simulink model "modeldefinitiu4t"  (Simulink 7.4)
settings: Solver=ode45  StartTime=t0  StopTime=t1  MaxStep=1e-4
values from neighbouring files (symbols this model uses):
  Ap = 90e3*sqrt(2)/sqrt(3)    [parametres.m]
  E0 = 145e3    (= 145000)    [parametres.m]
  f = 50    [parametres.m]
  ida3 = 0    [parametres.m]
  ida4 = 0    [parametres.m]
  it = [0 0.2 0.200001 0.35 0.3500001 t1]    [parametres.m]
  iv = [0 0 100e6 100e6 0 0]    [parametres.m]
  K3 = 1/20    (= 0.05)    [parametres.m]
  K4 = K3    (= 0.05)    [parametres.m]
  Ki = rl/tau    (= 1140.8)    [parametres.m]
  Kp = Ll/tau    (= 93)    [parametres.m]
  L1 = 0.005    [parametres.m]
  L2 = 0.0025    [parametres.m]
  L3 = 0.004    [parametres.m]
  Lac = 30e-3    (= 0.03)    [parametres.m]
  Ll = Lac    (= 0.03)    [parametres.m]
  Lx = 0.052*0.669    (= 0.034788)    [parametres.m]
  R1 = 0.5    [parametres.m]
  R2 = 0.25    [parametres.m]
  R3 = 0.4    [parametres.m]
  Rac = 3.68/10    (= 0.368)    [parametres.m]
  Rx = 4.8*0.669    (= 3.2112)    [parametres.m]
  sc = 0    [parametres.m]
  T = 1/12e3    (= 8.33333333333e-05)    [parametres.m]
undefined symbols (not defined in the file or in its folder): DiscIntNeverNeededParam
libraries: powerlib x62
(part 1 of 2)
settings Model: Creator=edu  LastModifiedBy=edu

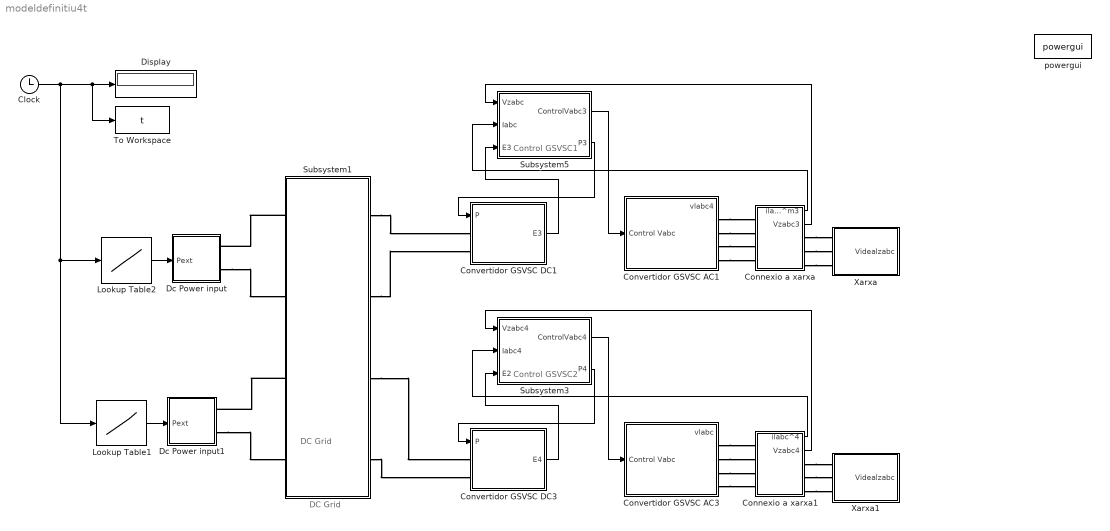
== system modeldefinitiu4t ==
  note: DC Grid
  note: Control GSVSC1
  note: DC Grid
  note: Control GSVSC2
  Clock : Clock
      settings: Decimation=10
  Connexio a xarxa : Subsystem
  Connexio a xarxa1 : Subsystem
  Convertidor GSVSC AC1 : Subsystem
  Convertidor GSVSC AC3 : Subsystem
  Convertidor GSVSC DC1 : Subsystem
  Convertidor GSVSC DC3 : Subsystem
  Dc Power input : Subsystem
  Dc Power input1 : Subsystem
  Display : Display
  Lookup Table1 : Lookup  InputValues=it  Table=iv  OutDataType=fixdt(1, 16)  OutScaling=2^0
  Lookup Table2 : Lookup  InputValues=it  Table=iv  OutDataType=fixdt(1, 16)  OutScaling=2^0
  Subsystem1 : Subsystem
  Subsystem3 : Subsystem
  Subsystem5 : Subsystem
  To Workspace : ToWorkspace  VariableName=t  SampleTime=T  SaveFormat=Array
  Xarxa : Subsystem
  Xarxa1 : Subsystem
  powergui : powerlib/powergui  SystemSampleTime=-1  SimulationMode=Continuous  SampleTime=50e-6  frequency=60  SPID=off  DisableSnubberDevices=off  DisableRonSwitches=off  DisableVfSwitches=off  SwTol=0  Interpol=off  frequencyindice=0  echomessages=off  HookPort=off  DisplayEquations=off  FunctionMessages=off  EnableUseOfTLC=off  x0status=blocks  RestoreLinks=warning  Frange=[0:2:500]  Ylog=off  Xlog=on  ShowGrid=off  save=off  variable=ZData  ZoomFFT=on  StartTime=0.0  cycles=1  DisplayStyle=1  fundamental=60  FreqAxis=off  MaxFrequency=1000  frequencyindicesteady=1  RmsSteady=1  display=off  Ts=0  methode=off
  wires:
  Clock/1 -> Display/1, To Workspace/1, Lookup Table2/1, Lookup Table1/1
  Lookup Table2/1 -> Dc Power input/1(Pext)
  Convertidor GSVSC DC1/1(E3) -> Subsystem5/3(E3)
  Subsystem5/1(ControlVabc3) -> Convertidor GSVSC AC1/1(Control Vabc)
  Connexio a xarxa/1(ilabc^m3) -> Subsystem5/2(Iabc)
  Subsystem5/2(P3) -> Convertidor GSVSC DC1/1(P)
  Connexio a xarxa/2(Vzabc3) -> Subsystem5/1(Vzabc)
  Lookup Table1/1 -> Dc Power input1/1(Pext)
  Convertidor GSVSC DC3/1(E4) -> Subsystem3/3(E2)
  Subsystem3/1(ControlVabc4) -> Convertidor GSVSC AC3/1(Control Vabc)
  Connexio a xarxa1/1(ilabc^4) -> Subsystem3/2(Iabc4)
  Subsystem3/2(P4) -> Convertidor GSVSC DC3/1(P)
  Connexio a xarxa1/2(Vzabc4) -> Subsystem3/1(Vzabc4)
  connections:
  Convertidor GSVSC AC1/RConn2 -- Connexio a xarxa/LConn2
  Connexio a xarxa/RConn1 -- Xarxa/LConn1
  Connexio a xarxa/RConn2 -- Xarxa/LConn2
  Connexio a xarxa/RConn3 -- Xarxa/LConn3
  Subsystem1/LConn1 -- Dc Power input/RConn1
  Dc Power input/RConn2 -- Subsystem1/LConn2
  Subsystem1/RConn2 -- Convertidor GSVSC DC1/LConn2
  Convertidor GSVSC AC1/RConn1 -- Connexio a xarxa/LConn1
  Convertidor GSVSC AC1/RConn3 -- Connexio a xarxa/LConn3
  Convertidor GSVSC AC1/RConn4 -- Connexio a xarxa/LConn4
  Convertidor GSVSC AC3/RConn4 -- Connexio a xarxa1/LConn4
  Convertidor GSVSC AC3/RConn3 -- Connexio a xarxa1/LConn3
  Convertidor GSVSC AC3/RConn1 -- Connexio a xarxa1/LConn1
  Subsystem1/RConn3 -- Convertidor GSVSC DC3/LConn1
  Subsystem1/LConn3 -- Dc Power input1/RConn1
  Connexio a xarxa1/RConn3 -- Xarxa1/LConn3
  Connexio a xarxa1/RConn2 -- Xarxa1/LConn2
  Connexio a xarxa1/RConn1 -- Xarxa1/LConn1
  Convertidor GSVSC AC3/RConn2 -- Connexio a xarxa1/LConn2
  Dc Power input1/RConn2 -- Subsystem1/LConn4
  Subsystem1/RConn4 -- Convertidor GSVSC DC3/LConn2
  Subsystem1/RConn1 -- Convertidor GSVSC DC1/LConn1

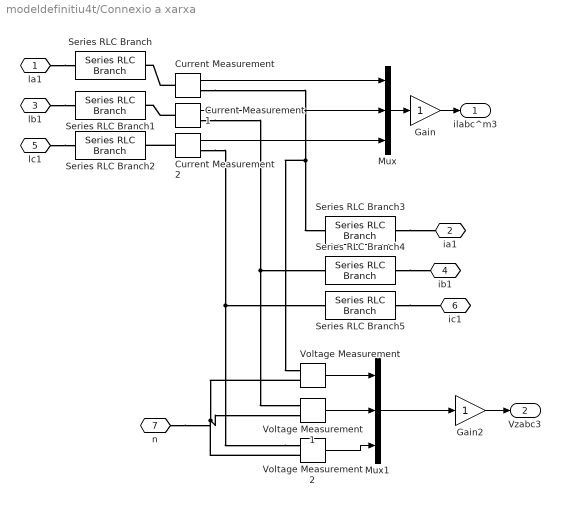
== system modeldefinitiu4t/Connexio a xarxa ==
  Current Measurement : powerlib/Measurements/Current Measurement  DialogController=POWERSYS.PowerSysDialog  SystemSampleTime=-1  PhasorSimulation=off  OutputType=Complex  PSBequivalent=0
  Current Measurement1 : powerlib/Measurements/Current Measurement  DialogController=POWERSYS.PowerSysDialog  SystemSampleTime=-1  PhasorSimulation=off  OutputType=Complex  PSBequivalent=0
  Current Measurement2 : powerlib/Measurements/Current Measurement  DialogController=POWERSYS.PowerSysDialog  SystemSampleTime=-1  PhasorSimulation=off  OutputType=Complex  PSBequivalent=0
  Gain : Gain  ParameterDataType=sfix(16)  ParameterScaling=2^0  OutDataType=sfix(16)  OutScaling=2^0  SampleTime=T
  Gain2 : Gain  ParameterDataType=sfix(16)  ParameterScaling=2^0  OutDataType=sfix(16)  OutScaling=2^0  SampleTime=T
  Mux : Mux  Inputs=3
  Mux1 : Mux  Inputs=3
  Series RLC Branch : powerlib/Elements/Series RLC Branch  DialogController=POWERSYS.PowerSysDialog  PhysicalDomain=powersysdomain  SubClassName=unknown  LeftPortType=p1  RightPortType=p1  LConnTagsString=__new0  RConnTagsString=__new0  BranchType=RL  Resistance=Rac  Inductance=Lac  SetiL0=off  InitialCurrent=0  Capacitance=1e-6  Setx0=off  InitialVoltage=0  Measurements=None
  Series RLC Branch1 : powerlib/Elements/Series RLC Branch  DialogController=POWERSYS.PowerSysDialog  PhysicalDomain=powersysdomain  SubClassName=unknown  LeftPortType=p1  RightPortType=p1  LConnTagsString=__new0  RConnTagsString=__new0  BranchType=RL  Resistance=Rac  Inductance=Lac  SetiL0=off  InitialCurrent=0  Capacitance=1e-6  Setx0=off  InitialVoltage=0  Measurements=None
  Series RLC Branch2 : powerlib/Elements/Series RLC Branch  DialogController=POWERSYS.PowerSysDialog  PhysicalDomain=powersysdomain  SubClassName=unknown  LeftPortType=p1  RightPortType=p1  LConnTagsString=__new0  RConnTagsString=__new0  BranchType=RL  Resistance=Rac  Inductance=Lac  SetiL0=off  InitialCurrent=0  Capacitance=1e-6  Setx0=off  InitialVoltage=0  Measurements=None
  Series RLC Branch3 : powerlib/Elements/Series RLC Branch  DialogController=POWERSYS.PowerSysDialog  PhysicalDomain=powersysdomain  SubClassName=unknown  LeftPortType=p1  RightPortType=p1  LConnTagsString=__new0  RConnTagsString=__new0  BranchType=RL  Resistance=Rx  Inductance=Lx  SetiL0=off  InitialCurrent=0  Capacitance=1e-6  Setx0=off  InitialVoltage=0  Measurements=None
  Series RLC Branch4 : powerlib/Elements/Series RLC Branch  DialogController=POWERSYS.PowerSysDialog  PhysicalDomain=powersysdomain  SubClassName=unknown  LeftPortType=p1  RightPortType=p1  LConnTagsString=__new0  RConnTagsString=__new0  BranchType=RL  Resistance=Rx  Inductance=Lx  SetiL0=off  InitialCurrent=0  Capacitance=1e-6  Setx0=off  InitialVoltage=0  Measurements=None
  Series RLC Branch5 : powerlib/Elements/Series RLC Branch  DialogController=POWERSYS.PowerSysDialog  PhysicalDomain=powersysdomain  SubClassName=unknown  LeftPortType=p1  RightPortType=p1  LConnTagsString=__new0  RConnTagsString=__new0  BranchType=RL  Resistance=Rx  Inductance=Lx  SetiL0=off  InitialCurrent=0  Capacitance=1e-6  Setx0=off  InitialVoltage=0  Measurements=None
  Voltage Measurement : powerlib/Measurements/Voltage Measurement  DialogController=POWERSYS.PowerSysDialog  SystemSampleTime=-1  PhasorSimulation=off  OutputType=Complex  PSBequivalent=0
  Voltage Measurement1 : powerlib/Measurements/Voltage Measurement  DialogController=POWERSYS.PowerSysDialog  SystemSampleTime=-1  PhasorSimulation=off  OutputType=Complex  PSBequivalent=0
  Voltage Measurement2 : powerlib/Measurements/Voltage Measurement  DialogController=POWERSYS.PowerSysDialog  SystemSampleTime=-1  PhasorSimulation=off  OutputType=Complex  PSBequivalent=0
  la1 : PMIOPort  Port=1  Side=Left
  ia1 : PMIOPort  Port=2  Side=Right
  lb1 : PMIOPort  Port=3  Side=Left
  ib1 : PMIOPort  Port=4  Side=Right
  lc1 : PMIOPort  Port=5  Side=Left
  ic1 : PMIOPort  Port=6  Side=Right
  n : PMIOPort  Port=7  Side=Left
  ilabc^m3 : Outport  OutDataType=sfix(16)  OutScaling=2^0
  Vzabc3 : Outport  Port=2
  wires:
  Current Measurement/1 -> Mux/1
  Current Measurement1/1 -> Mux/2
  Current Measurement2/1 -> Mux/3
  Mux/1 -> Gain/1
  Gain/1 -> ilabc^m3/1
  Gain2/1 -> Vzabc3/1
  Voltage Measurement/1 -> Mux1/1
  Voltage Measurement1/1 -> Mux1/2
  Voltage Measurement2/1 -> Mux1/3
  Mux1/1 -> Gain2/1
  connections:
  la1/RConn1 -- Series RLC Branch/LConn1
  Current Measurement/LConn1 -- Series RLC Branch/RConn1
  lb1/RConn1 -- Series RLC Branch1/LConn1
  Current Measurement1/LConn1 -- Series RLC Branch1/RConn1
  lc1/RConn1 -- Series RLC Branch2/LConn1
  Current Measurement2/LConn1 -- Series RLC Branch2/RConn1
  Voltage Measurement2/LConn1 -- Current Measurement2/RConn1 -- Series RLC Branch5/LConn1
  Current Measurement1/RConn1 -- Series RLC Branch4/LConn1 -- Voltage Measurement1/LConn1
  Current Measurement/RConn1 -- Series RLC Branch3/LConn1 -- Voltage Measurement/LConn1
  Series RLC Branch3/RConn1 -- ia1/RConn1
  Series RLC Branch4/RConn1 -- ib1/RConn1
  Series RLC Branch5/RConn1 -- ic1/RConn1
  Voltage Measurement2/LConn2 -- Voltage Measurement/LConn2 -- Voltage Measurement1/LConn2 -- n/RConn1

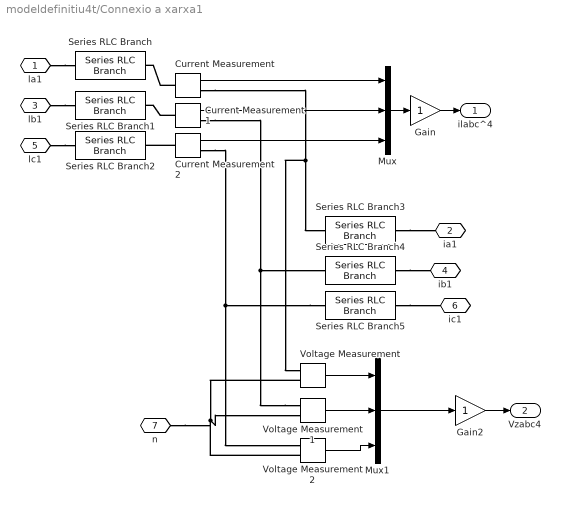
== system modeldefinitiu4t/Connexio a xarxa1 ==
  Current Measurement : powerlib/Measurements/Current Measurement  DialogController=POWERSYS.PowerSysDialog  SystemSampleTime=-1  PhasorSimulation=off  OutputType=Complex  PSBequivalent=0
  Current Measurement1 : powerlib/Measurements/Current Measurement  DialogController=POWERSYS.PowerSysDialog  SystemSampleTime=-1  PhasorSimulation=off  OutputType=Complex  PSBequivalent=0
  Current Measurement2 : powerlib/Measurements/Current Measurement  DialogController=POWERSYS.PowerSysDialog  SystemSampleTime=-1  PhasorSimulation=off  OutputType=Complex  PSBequivalent=0
  Gain : Gain  ParameterDataType=sfix(16)  ParameterScaling=2^0  OutDataType=sfix(16)  OutScaling=2^0  SampleTime=T
  Gain2 : Gain  ParameterDataType=sfix(16)  ParameterScaling=2^0  OutDataType=sfix(16)  OutScaling=2^0  SampleTime=T
  Mux : Mux  Inputs=3
  Mux1 : Mux  Inputs=3
  Series RLC Branch : powerlib/Elements/Series RLC Branch  DialogController=POWERSYS.PowerSysDialog  PhysicalDomain=powersysdomain  SubClassName=unknown  LeftPortType=p1  RightPortType=p1  LConnTagsString=__new0  RConnTagsString=__new0  BranchType=RL  Resistance=Rac  Inductance=Lac  SetiL0=off  InitialCurrent=0  Capacitance=1e-6  Setx0=off  InitialVoltage=0  Measurements=None
  Series RLC Branch1 : powerlib/Elements/Series RLC Branch  DialogController=POWERSYS.PowerSysDialog  PhysicalDomain=powersysdomain  SubClassName=unknown  LeftPortType=p1  RightPortType=p1  LConnTagsString=__new0  RConnTagsString=__new0  BranchType=RL  Resistance=Rac  Inductance=Lac  SetiL0=off  InitialCurrent=0  Capacitance=1e-6  Setx0=off  InitialVoltage=0  Measurements=None
  Series RLC Branch2 : powerlib/Elements/Series RLC Branch  DialogController=POWERSYS.PowerSysDialog  PhysicalDomain=powersysdomain  SubClassName=unknown  LeftPortType=p1  RightPortType=p1  LConnTagsString=__new0  RConnTagsString=__new0  BranchType=RL  Resistance=Rac  Inductance=Lac  SetiL0=off  InitialCurrent=0  Capacitance=1e-6  Setx0=off  InitialVoltage=0  Measurements=None
  Series RLC Branch3 : powerlib/Elements/Series RLC Branch  DialogController=POWERSYS.PowerSysDialog  PhysicalDomain=powersysdomain  SubClassName=unknown  LeftPortType=p1  RightPortType=p1  LConnTagsString=__new0  RConnTagsString=__new0  BranchType=RL  Resistance=Rx  Inductance=Lx  SetiL0=off  InitialCurrent=0  Capacitance=1e-6  Setx0=off  InitialVoltage=0  Measurements=None
  Series RLC Branch4 : powerlib/Elements/Series RLC Branch  DialogController=POWERSYS.PowerSysDialog  PhysicalDomain=powersysdomain  SubClassName=unknown  LeftPortType=p1  RightPortType=p1  LConnTagsString=__new0  RConnTagsString=__new0  BranchType=RL  Resistance=Rx  Inductance=Lx  SetiL0=off  InitialCurrent=0  Capacitance=1e-6  Setx0=off  InitialVoltage=0  Measurements=None
  Series RLC Branch5 : powerlib/Elements/Series RLC Branch  DialogController=POWERSYS.PowerSysDialog  PhysicalDomain=powersysdomain  SubClassName=unknown  LeftPortType=p1  RightPortType=p1  LConnTagsString=__new0  RConnTagsString=__new0  BranchType=RL  Resistance=Rx  Inductance=Lx  SetiL0=off  InitialCurrent=0  Capacitance=1e-6  Setx0=off  InitialVoltage=0  Measurements=None
  Voltage Measurement : powerlib/Measurements/Voltage Measurement  DialogController=POWERSYS.PowerSysDialog  SystemSampleTime=-1  PhasorSimulation=off  OutputType=Complex  PSBequivalent=0
  Voltage Measurement1 : powerlib/Measurements/Voltage Measurement  DialogController=POWERSYS.PowerSysDialog  SystemSampleTime=-1  PhasorSimulation=off  OutputType=Complex  PSBequivalent=0
  Voltage Measurement2 : powerlib/Measurements/Voltage Measurement  DialogController=POWERSYS.PowerSysDialog  SystemSampleTime=-1  PhasorSimulation=off  OutputType=Complex  PSBequivalent=0
  la1 : PMIOPort  Port=1  Side=Left
  ia1 : PMIOPort  Port=2  Side=Right
  lb1 : PMIOPort  Port=3  Side=Left
  ib1 : PMIOPort  Port=4  Side=Right
  lc1 : PMIOPort  Port=5  Side=Left
  ic1 : PMIOPort  Port=6  Side=Right
  n : PMIOPort  Port=7  Side=Left
  ilabc^4 : Outport  OutDataType=sfix(16)  OutScaling=2^0
  Vzabc4 : Outport  Port=2
  wires:
  Mux1/1 -> Gain2/1
  Voltage Measurement2/1 -> Mux1/3
  Voltage Measurement1/1 -> Mux1/2
  Voltage Measurement/1 -> Mux1/1
  Gain2/1 -> Vzabc4/1
  Gain/1 -> ilabc^4/1
  Mux/1 -> Gain/1
  Current Measurement2/1 -> Mux/3
  Current Measurement1/1 -> Mux/2
  Current Measurement/1 -> Mux/1
  connections:
  n/RConn1 -- Voltage Measurement1/LConn2 -- Voltage Measurement/LConn2 -- Voltage Measurement2/LConn2
  Series RLC Branch5/RConn1 -- ic1/RConn1
  Series RLC Branch4/RConn1 -- ib1/RConn1
  Series RLC Branch3/RConn1 -- ia1/RConn1
  Voltage Measurement/LConn1 -- Series RLC Branch3/LConn1 -- Current Measurement/RConn1
  Voltage Measurement1/LConn1 -- Series RLC Branch4/LConn1 -- Current Measurement1/RConn1
  Series RLC Branch5/LConn1 -- Current Measurement2/RConn1 -- Voltage Measurement2/LConn1
  Current Measurement2/LConn1 -- Series RLC Branch2/RConn1
  lc1/RConn1 -- Series RLC Branch2/LConn1
  Current Measurement1/LConn1 -- Series RLC Branch1/RConn1
  lb1/RConn1 -- Series RLC Branch1/LConn1
  Current Measurement/LConn1 -- Series RLC Branch/RConn1
  la1/RConn1 -- Series RLC Branch/LConn1

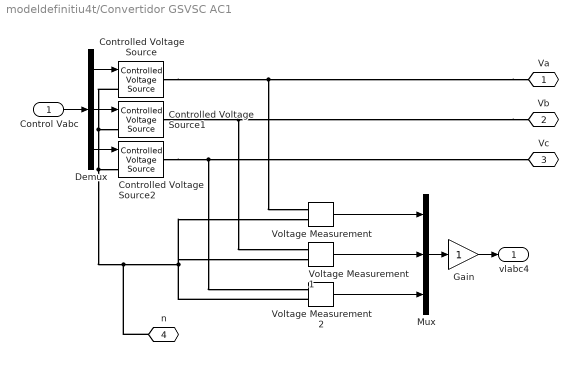
== system modeldefinitiu4t/Convertidor GSVSC AC1 ==
  Control Vabc : Inport
  Controlled Voltage Source : powerlib/Electrical Sources/Controlled Voltage Source  DialogController=POWERSYS.PowerSysDialog  SystemSampleTime=-1  Initialize=on  Source_Type=AC  Amplitude=0  Phase=0  Frequency=0  Measurements=None
  Controlled Voltage Source1 : powerlib/Electrical Sources/Controlled Voltage Source  DialogController=POWERSYS.PowerSysDialog  SystemSampleTime=-1  Initialize=on  Source_Type=AC  Amplitude=0  Phase=0  Frequency=0  Measurements=None
  Controlled Voltage Source2 : powerlib/Electrical Sources/Controlled Voltage Source  DialogController=POWERSYS.PowerSysDialog  SystemSampleTime=-1  Initialize=on  Source_Type=AC  Amplitude=0  Phase=0  Frequency=0  Measurements=None
  Demux : Demux  Outputs=3
  Gain : Gain  ParameterDataType=sfix(16)  ParameterScaling=2^0  OutDataType=sfix(16)  OutScaling=2^0  SampleTime=T
  Mux : Mux  Inputs=3
  Voltage Measurement : powerlib/Measurements/Voltage Measurement  DialogController=POWERSYS.PowerSysDialog  SystemSampleTime=-1  PhasorSimulation=off  OutputType=Complex  PSBequivalent=0
  Voltage Measurement1 : powerlib/Measurements/Voltage Measurement  DialogController=POWERSYS.PowerSysDialog  SystemSampleTime=-1  PhasorSimulation=off  OutputType=Complex  PSBequivalent=0
  Voltage Measurement2 : powerlib/Measurements/Voltage Measurement  DialogController=POWERSYS.PowerSysDialog  SystemSampleTime=-1  PhasorSimulation=off  OutputType=Complex  PSBequivalent=0
  Va : PMIOPort  Port=1  Side=Right
  Vb : PMIOPort  Port=2  Side=Right
  Vc : PMIOPort  Port=3  Side=Right
  n : PMIOPort  Port=4  Side=Right
  vlabc4 : Outport
  wires:
  Demux/3 -> Controlled Voltage Source2/1
  Demux/2 -> Controlled Voltage Source1/1
  Demux/1 -> Controlled Voltage Source/1
  Voltage Measurement/1 -> Mux/1
  Voltage Measurement1/1 -> Mux/2
  Voltage Measurement2/1 -> Mux/3
  Mux/1 -> Gain/1
  Gain/1 -> vlabc4/1
  Control Vabc/1 -> Demux/1
  connections:
  Va/RConn1 -- Controlled Voltage Source/RConn1 -- Voltage Measurement/LConn1
  Vb/RConn1 -- Controlled Voltage Source1/RConn1 -- Voltage Measurement1/LConn1
  Controlled Voltage Source2/RConn1 -- Vc/RConn1 -- Voltage Measurement2/LConn1
  Controlled Voltage Source/LConn1 -- Controlled Voltage Source1/LConn1 -- Controlled Voltage Source2/LConn1 -- Voltage Measurement2/LConn2 -- Voltage Measurement/LConn2 -- Voltage Measurement1/LConn2 -- n/RConn1

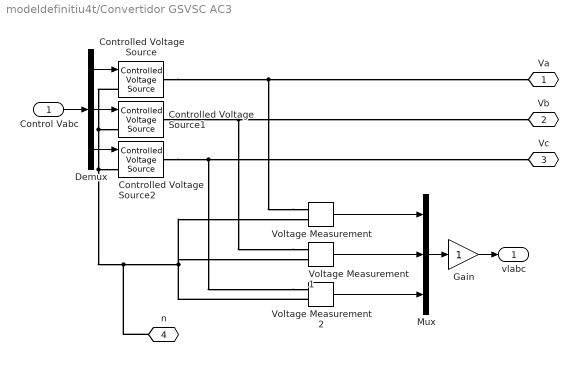
== system modeldefinitiu4t/Convertidor GSVSC AC3 ==
  Control Vabc : Inport
  Controlled Voltage Source : powerlib/Electrical Sources/Controlled Voltage Source  DialogController=POWERSYS.PowerSysDialog  SystemSampleTime=-1  Initialize=on  Source_Type=AC  Amplitude=0  Phase=0  Frequency=0  Measurements=None
  Controlled Voltage Source1 : powerlib/Electrical Sources/Controlled Voltage Source  DialogController=POWERSYS.PowerSysDialog  SystemSampleTime=-1  Initialize=on  Source_Type=AC  Amplitude=0  Phase=0  Frequency=0  Measurements=None
  Controlled Voltage Source2 : powerlib/Electrical Sources/Controlled Voltage Source  DialogController=POWERSYS.PowerSysDialog  SystemSampleTime=-1  Initialize=on  Source_Type=AC  Amplitude=0  Phase=0  Frequency=0  Measurements=None
  Demux : Demux  Outputs=3
  Gain : Gain  ParameterDataType=sfix(16)  ParameterScaling=2^0  OutDataType=sfix(16)  OutScaling=2^0  SampleTime=T
  Mux : Mux  Inputs=3
  Voltage Measurement : powerlib/Measurements/Voltage Measurement  DialogController=POWERSYS.PowerSysDialog  SystemSampleTime=-1  PhasorSimulation=off  OutputType=Complex  PSBequivalent=0
  Voltage Measurement1 : powerlib/Measurements/Voltage Measurement  DialogController=POWERSYS.PowerSysDialog  SystemSampleTime=-1  PhasorSimulation=off  OutputType=Complex  PSBequivalent=0
  Voltage Measurement2 : powerlib/Measurements/Voltage Measurement  DialogController=POWERSYS.PowerSysDialog  SystemSampleTime=-1  PhasorSimulation=off  OutputType=Complex  PSBequivalent=0
  Va : PMIOPort  Port=1  Side=Right
  Vb : PMIOPort  Port=2  Side=Right
  Vc : PMIOPort  Port=3  Side=Right
  n : PMIOPort  Port=4  Side=Right
  vlabc : Outport
  wires:
  Control Vabc/1 -> Demux/1
  Gain/1 -> vlabc/1
  Mux/1 -> Gain/1
  Voltage Measurement2/1 -> Mux/3
  Voltage Measurement1/1 -> Mux/2
  Voltage Measurement/1 -> Mux/1
  Demux/1 -> Controlled Voltage Source/1
  Demux/2 -> Controlled Voltage Source1/1
  Demux/3 -> Controlled Voltage Source2/1
  connections:
  n/RConn1 -- Voltage Measurement1/LConn2 -- Voltage Measurement/LConn2 -- Voltage Measurement2/LConn2 -- Controlled Voltage Source2/LConn1 -- Controlled Voltage Source1/LConn1 -- Controlled Voltage Source/LConn1
  Voltage Measurement2/LConn1 -- Vc/RConn1 -- Controlled Voltage Source2/RConn1
  Voltage Measurement1/LConn1 -- Controlled Voltage Source1/RConn1 -- Vb/RConn1
  Voltage Measurement/LConn1 -- Controlled Voltage Source/RConn1 -- Va/RConn1

== system modeldefinitiu4t/Convertidor GSVSC DC1 ==
  P : Inport
  Controlled Current Source1 : powerlib/Electrical Sources/Controlled Current Source  DialogController=POWERSYS.PowerSysDialog  SystemSampleTime=-1  Initialize=on  Source_Type=DC  Amplitude=10  Phase=0  Frequency=0  Measurements=None
  Current Measurement1 : powerlib/Measurements/Current Measurement  DialogController=POWERSYS.PowerSysDialog  SystemSampleTime=-1  PhasorSimulation=off  OutputType=Complex  PSBequivalent=0
  Divide : Product  Inputs=/*  OutDataType=fixdt(1, 16)  OutScaling=2^-10
  Gain1 : Gain  ParameterDataType=sfix(16)  ParameterScaling=2^0  OutDataType=sfix(16)  OutScaling=2^0  SampleTime=T
  Gain2 : Gain  ParameterDataType=sfix(16)  ParameterScaling=2^0  OutDataType=sfix(16)  OutScaling=2^0  SampleTime=T
  Scope : Scope
      settings: YMin=-100  YMax=700
  To Workspace1 : ToWorkspace  VariableName=i3  SampleTime=-1  SaveFormat=Array
  To Workspace2 : ToWorkspace  VariableName=E3  SampleTime=-1  SaveFormat=Array
  Voltage Measurement : powerlib/Measurements/Voltage Measurement  DialogController=POWERSYS.PowerSysDialog  SystemSampleTime=-1  PhasorSimulation=off  OutputType=Complex  PSBequivalent=0
  Idc+ : PMIOPort  Port=1  Side=Left
  idc- : PMIOPort  Port=2  Side=Left
  E3 : Outport
  wires:
  Voltage Measurement/1 -> E3/1, Divide/1, Gain1/1
  Divide/1 -> Controlled Current Source1/1
  Current Measurement1/1 -> Gain2/1
  P/1 -> Divide/2
  Gain1/1 -> To Workspace2/1
  Gain2/1 -> To Workspace1/1, Scope/1
  connections:
  Idc+/RConn1 -- Controlled Current Source1/LConn1 -- Voltage Measurement/LConn1
  Current Measurement1/LConn1 -- Controlled Current Source1/RConn1
  Current Measurement1/RConn1 -- idc-/RConn1 -- Voltage Measurement/LConn2

== system modeldefinitiu4t/Convertidor GSVSC DC3 ==
  P : Inport
  Controlled Current Source1 : powerlib/Electrical Sources/Controlled Current Source  DialogController=POWERSYS.PowerSysDialog  SystemSampleTime=-1  Initialize=on  Source_Type=DC  Amplitude=10  Phase=0  Frequency=0  Measurements=None
  Current Measurement1 : powerlib/Measurements/Current Measurement  DialogController=POWERSYS.PowerSysDialog  SystemSampleTime=-1  PhasorSimulation=off  OutputType=Complex  PSBequivalent=0
  Divide : Product  Inputs=/*  OutDataType=fixdt(1, 16)  OutScaling=2^-10
  Gain1 : Gain  ParameterDataType=sfix(16)  ParameterScaling=2^0  OutDataType=sfix(16)  OutScaling=2^0  SampleTime=T
  Gain2 : Gain  ParameterDataType=sfix(16)  ParameterScaling=2^0  OutDataType=sfix(16)  OutScaling=2^0  SampleTime=T
  Scope : Scope
      settings: YMin=-100  YMax=700
  To Workspace1 : ToWorkspace  VariableName=i4  SampleTime=-1  SaveFormat=Array
  To Workspace2 : ToWorkspace  VariableName=E4  SampleTime=-1  SaveFormat=Array
  Voltage Measurement : powerlib/Measurements/Voltage Measurement  DialogController=POWERSYS.PowerSysDialog  SystemSampleTime=-1  PhasorSimulation=off  OutputType=Complex  PSBequivalent=0
  Idc+ : PMIOPort  Port=1  Side=Left
  idc- : PMIOPort  Port=2  Side=Left
  E4 : Outport
  wires:
  Gain2/1 -> Scope/1, To Workspace1/1
  Gain1/1 -> To Workspace2/1
  P/1 -> Divide/2
  Current Measurement1/1 -> Gain2/1
  Divide/1 -> Controlled Current Source1/1
  Voltage Measurement/1 -> Gain1/1, Divide/1, E4/1
  connections:
  Voltage Measurement/LConn2 -- idc-/RConn1 -- Current Measurement1/RConn1
  Current Measurement1/LConn1 -- Controlled Current Source1/RConn1
  Voltage Measurement/LConn1 -- Controlled Current Source1/LConn1 -- Idc+/RConn1

== system modeldefinitiu4t/Dc Power input ==
  Pext : Inport
  Controlled Current Source2 : powerlib/Electrical Sources/Controlled Current Source  DialogController=POWERSYS.PowerSysDialog  SystemSampleTime=-1  Initialize=on  Source_Type=DC  Amplitude=10  Phase=0  Frequency=0  Measurements=None
  Current Measurement1 : powerlib/Measurements/Current Measurement  DialogController=POWERSYS.PowerSysDialog  SystemSampleTime=-1  PhasorSimulation=off  OutputType=Complex  PSBequivalent=0
  Divide1 : Product  Inputs=*/  OutDataType=fixdt(1, 16)  OutScaling=2^-10
  Gain1 : Gain  ParameterDataType=sfix(16)  ParameterScaling=2^0  OutDataType=sfix(16)  OutScaling=2^0  SampleTime=T
  Gain2 : Gain  ParameterDataType=sfix(16)  ParameterScaling=2^0  OutDataType=sfix(16)  OutScaling=2^0  SampleTime=T
  Gain3 : Gain  ParameterDataType=sfix(16)  ParameterScaling=2^0  OutDataType=sfix(16)  OutScaling=2^0  SampleTime=T
  To Workspace1 : ToWorkspace  VariableName=E1  SampleTime=-1  SaveFormat=Array
  To Workspace2 : ToWorkspace  VariableName=Pin1  SampleTime=-1  SaveFormat=Array
  To Workspace3 : ToWorkspace  VariableName=i1  SampleTime=-1  SaveFormat=Array
  Voltage Measurement1 : powerlib/Measurements/Voltage Measurement  DialogController=POWERSYS.PowerSysDialog  SystemSampleTime=-1  PhasorSimulation=off  OutputType=Complex  PSBequivalent=0
  Idc+ : PMIOPort  Port=1  Side=Right
  Idc- : PMIOPort  Port=2  Side=Right
  wires:
  Voltage Measurement1/1 -> Divide1/2, Gain1/1
  Divide1/1 -> Controlled Current Source2/1
  Pext/1 -> Divide1/1, Gain3/1
  Current Measurement1/1 -> Gain2/1
  Gain2/1 -> To Workspace3/1
  Gain1/1 -> To Workspace1/1
  Gain3/1 -> To Workspace2/1
  connections:
  Idc-/RConn1 -- Controlled Current Source2/LConn1 -- Voltage Measurement1/LConn2
  Current Measurement1/LConn1 -- Controlled Current Source2/RConn1 -- Voltage Measurement1/LConn1
  Current Measurement1/RConn1 -- Idc+/RConn1

== system modeldefinitiu4t/Dc Power input1 ==
  Pext : Inport
  Controlled Current Source2 : powerlib/Electrical Sources/Controlled Current Source  DialogController=POWERSYS.PowerSysDialog  SystemSampleTime=-1  Initialize=on  Source_Type=DC  Amplitude=10  Phase=0  Frequency=0  Measurements=None
  Current Measurement1 : powerlib/Measurements/Current Measurement  DialogController=POWERSYS.PowerSysDialog  SystemSampleTime=-1  PhasorSimulation=off  OutputType=Complex  PSBequivalent=0
  Divide1 : Product  Inputs=*/  OutDataType=fixdt(1, 16)  OutScaling=2^-10
  Gain1 : Gain  ParameterDataType=sfix(16)  ParameterScaling=2^0  OutDataType=sfix(16)  OutScaling=2^0  SampleTime=T
  Gain2 : Gain  ParameterDataType=sfix(16)  ParameterScaling=2^0  OutDataType=sfix(16)  OutScaling=2^0  SampleTime=T
  Gain3 : Gain  ParameterDataType=sfix(16)  ParameterScaling=2^0  OutDataType=sfix(16)  OutScaling=2^0  SampleTime=T
  To Workspace1 : ToWorkspace  VariableName=E2  SampleTime=-1  SaveFormat=Array
  To Workspace2 : ToWorkspace  VariableName=Pin2  SampleTime=-1  SaveFormat=Array
  To Workspace3 : ToWorkspace  VariableName=i2  SampleTime=-1  SaveFormat=Array
  Voltage Measurement1 : powerlib/Measurements/Voltage Measurement  DialogController=POWERSYS.PowerSysDialog  SystemSampleTime=-1  PhasorSimulation=off  OutputType=Complex  PSBequivalent=0
  Idc+ : PMIOPort  Port=1  Side=Right
  Idc- : PMIOPort  Port=2  Side=Right
  wires:
  Gain3/1 -> To Workspace2/1
  Gain1/1 -> To Workspace1/1
  Gain2/1 -> To Workspace3/1
  Current Measurement1/1 -> Gain2/1
  Pext/1 -> Gain3/1, Divide1/1
  Divide1/1 -> Controlled Current Source2/1
  Voltage Measurement1/1 -> Gain1/1, Divide1/2
  connections:
  Current Measurement1/RConn1 -- Idc+/RConn1
  Voltage Measurement1/LConn1 -- Controlled Current Source2/RConn1 -- Current Measurement1/LConn1
  Voltage Measurement1/LConn2 -- Controlled Current Source2/LConn1 -- Idc-/RConn1

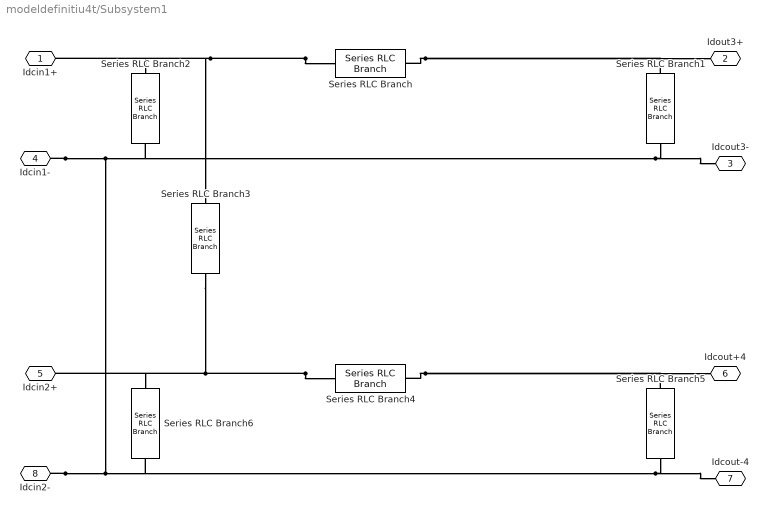
== system modeldefinitiu4t/Subsystem1 ==
  Series RLC Branch : powerlib/Elements/Series RLC Branch  DialogController=POWERSYS.PowerSysDialog  PhysicalDomain=powersysdomain  SubClassName=unknown  LeftPortType=p1  RightPortType=p1  LConnTagsString=__new0  RConnTagsString=__new0  BranchType=RL  Resistance=R1  Inductance=L1  SetiL0=off  InitialCurrent=0  Capacitance=1e-6  Setx0=off  InitialVoltage=0  Measurements=None
  Series RLC Branch{1..2,5..6} (4 alike) : powerlib/Elements/Series RLC Branch  DialogController=POWERSYS.PowerSysDialog  PhysicalDomain=powersysdomain  SubClassName=unknown  LeftPortType=p1  RightPortType=p1  LConnTagsString=__new0  RConnTagsString=__new0  BranchType=C  Resistance=1.0  Inductance=1.0  SetiL0=off  InitialCurrent=0  Capacitance=150e-6  Setx0=on  InitialVoltage=150e3  Measurements=None
  Series RLC Branch3 : powerlib/Elements/Series RLC Branch  DialogController=POWERSYS.PowerSysDialog  PhysicalDomain=powersysdomain  SubClassName=unknown  LeftPortType=p1  RightPortType=p1  LConnTagsString=__new0  RConnTagsString=__new0  BranchType=RL  Resistance=R2  Inductance=L2  SetiL0=off  InitialCurrent=0  Capacitance=1e-6  Setx0=off  InitialVoltage=0  Measurements=None
  Series RLC Branch4 : powerlib/Elements/Series RLC Branch  DialogController=POWERSYS.PowerSysDialog  PhysicalDomain=powersysdomain  SubClassName=unknown  LeftPortType=p1  RightPortType=p1  LConnTagsString=__new0  RConnTagsString=__new0  BranchType=RL  Resistance=R3  Inductance=L3  SetiL0=off  InitialCurrent=0  Capacitance=1e-6  Setx0=off  InitialVoltage=0  Measurements=None
  Idcin1+ : PMIOPort  Port=1  Side=Left
  Idout3+ : PMIOPort  Port=2  Side=Right
  Idcout3- : PMIOPort  Port=3  Side=Right
  Idcin1- : PMIOPort  Port=4  Side=Left
  Idcin2+ : PMIOPort  Port=5  Side=Left
  Idcout+4 : PMIOPort  Port=6  Side=Right
  Idcout-4 : PMIOPort  Port=7  Side=Right
  Idcin2- : PMIOPort  Port=8  Side=Left
  connections:
  Idcin1+/RConn1 -- Series RLC Branch/LConn1 -- Series RLC Branch2/LConn1 -- Series RLC Branch3/LConn1
  Series RLC Branch/RConn1 -- Series RLC Branch1/LConn1 -- Idout3+/RConn1
  Idcin1-/RConn1 -- Series RLC Branch1/RConn1 -- Idcout3-/RConn1 -- Series RLC Branch2/RConn1 -- Series RLC Branch6/RConn1 -- Idcin2-/RConn1 -- Idcout-4/RConn1 -- Series RLC Branch5/RConn1
  Series RLC Branch4/LConn1 -- Series RLC Branch6/LConn1 -- Idcin2+/RConn1 -- Series RLC Branch3/RConn1
  Series RLC Branch4/RConn1 -- Idcout+4/RConn1 -- Series RLC Branch5/LConn1

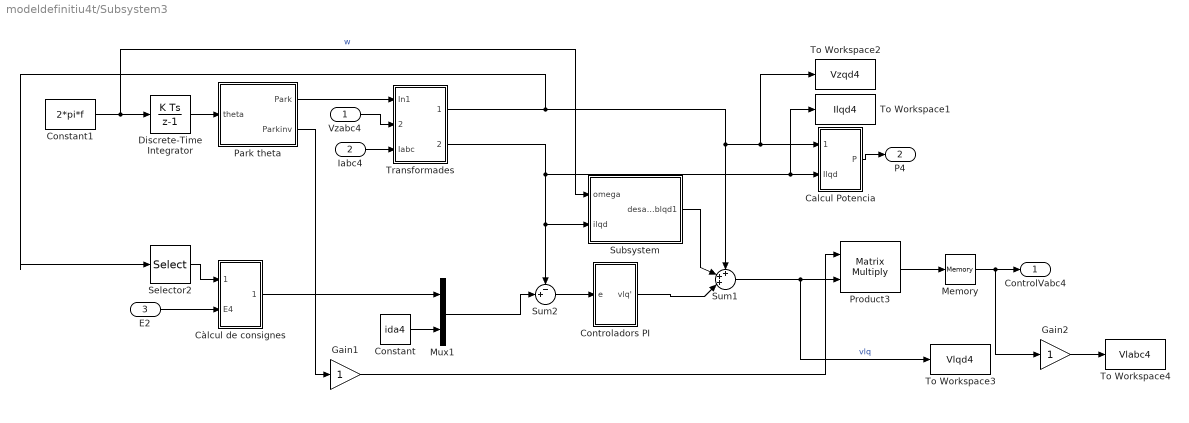
== system modeldefinitiu4t/Subsystem3 ==
  Vzabc4 : Inport
  Iabc4 : Inport  Port=2
  E2 : Inport  Port=3  OutDataType=fixdt(1, 16)  OutScaling=2^0
  Calcul Potencia : Subsystem
  Constant : Constant  Value=ida4  OutDataType=fixdt(1, 16)  OutScaling=2^0
  Constant1 : Constant  Value=2*pi*f  OutDataType=sfix(16)  OutScaling=2^0  SampleTime=T
  Controladors PI : Subsystem
  Càlcul de consignes : Subsystem
  Discrete-Time Integrator : DiscreteIntegrator  SampleTime=T  OutDataType=sfix(16)  OutScaling=2^0  ICPrevOutput=DiscIntNeverNeededParam  ICPrevScaledInput=DiscIntNeverNeededParam
  Gain1 : Gain  ParameterDataType=sfix(16)  ParameterScaling=2^0  OutDataType=sfix(16)  OutScaling=2^0  SampleTime=T
  Gain2 : Gain  ParameterDataType=sfix(16)  ParameterScaling=2^0  OutDataType=sfix(16)  OutScaling=2^0  SampleTime=T
  Memory : Memory
  Mux1 : Mux  Inputs=2
  Park theta : Subsystem
  Product3 : Product  Multiplication=Matrix(*)  OutDataType=sfix(16)  OutScaling=2^0  RndMeth=Zero
  Selector2 : Selector  InputPortWidth=2  IndexOptions=Index vector (dialog)  Indices=[1]  OutputSizes=1
  Subsystem : Subsystem
  Sum1 : Sum  Inputs=+++|  OutDataType=sfix(16)  OutScaling=2^0
  Sum2 : Sum  Inputs=-+|  OutDataType=sfix(16)  OutScaling=2^0
  To Workspace1 : ToWorkspace  VariableName=Ilqd4  SampleTime=-1  SaveFormat=Array
  To Workspace2 : ToWorkspace  VariableName=Vzqd4  SampleTime=-1  SaveFormat=Array
  To Workspace3 : ToWorkspace  VariableName=Vlqd4  SampleTime=-1  SaveFormat=Array
  To Workspace4 : ToWorkspace  VariableName=Vlabc4  SampleTime=-1  SaveFormat=Array
  Transformades : Subsystem
  ControlVabc4 : Outport
  P4 : Outport  Port=2
  wires:
  Gain2/1 -> To Workspace4/1
  Iabc4/1 -> Transformades/3(Iabc)
  Vzabc4/1 -> Transformades/2(Vzabc)
  Controladors PI/1(vlq') -> Sum1/3
  Transformades/1(Vzqd4) -> To Workspace2/1, Calcul Potencia/1(Vzqd), Sum1/1, Selector2/1
  Selector2/1 -> Càlcul de consignes/1(vzq4)
  Càlcul de consignes/1(iqa4) -> Mux1/1
  Constant/1 -> Mux1/2
  E2/1 -> Càlcul de consignes/2(E4)
  Mux1/1 -> Sum2/2
  Transformades/2(Iqd4) -> To Workspace1/1, Calcul Potencia/2(Ilqd), Subsystem/2(ilqd), Sum2/1
  Calcul Potencia/1(P) -> P4/1
  Memory/1 -> Gain2/1, ControlVabc4/1
  Sum1/1 -> To Workspace3/1, Product3/2  "vlq"
  Gain1/1 -> Product3/1
  Product3/1 -> Memory/1
  Subsystem/1(desacoblqd1) -> Sum1/2
  Sum2/1 -> Controladors PI/1(e)
  Park theta/2(Parkinv) -> Gain1/1
  Park theta/1(Park) -> Transformades/1(In1)
  Discrete-Time Integrator/1 -> Park theta/1(theta)
  Constant1/1 -> Subsystem/1(omega), Discrete-Time Integrator/1  "w"

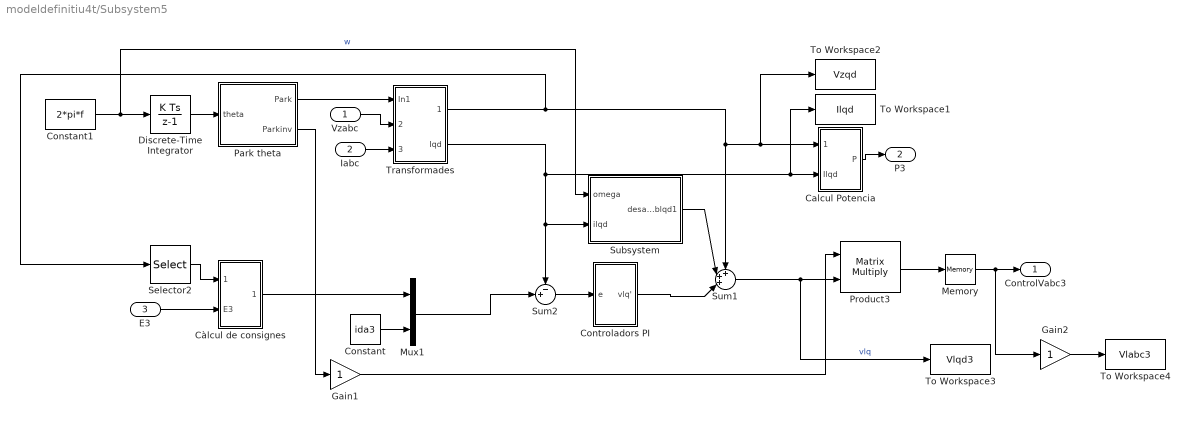
== system modeldefinitiu4t/Subsystem5 ==
  Vzabc : Inport
  Iabc : Inport  Port=2
  E3 : Inport  Port=3  OutDataType=fixdt(1, 16)  OutScaling=2^0
  Calcul Potencia : Subsystem
  Constant : Constant  Value=ida3  OutDataType=fixdt(1, 16)  OutScaling=2^0
  Constant1 : Constant  Value=2*pi*f  OutDataType=sfix(16)  OutScaling=2^0  SampleTime=T
  Controladors PI : Subsystem
  Càlcul de consignes : Subsystem
  Discrete-Time Integrator : DiscreteIntegrator  SampleTime=T  OutDataType=sfix(16)  OutScaling=2^0  ICPrevOutput=DiscIntNeverNeededParam  ICPrevScaledInput=DiscIntNeverNeededParam
  Gain1 : Gain  ParameterDataType=sfix(16)  ParameterScaling=2^0  OutDataType=sfix(16)  OutScaling=2^0  SampleTime=T
  Gain2 : Gain  ParameterDataType=sfix(16)  ParameterScaling=2^0  OutDataType=sfix(16)  OutScaling=2^0  SampleTime=T
  Memory : Memory
  Mux1 : Mux  Inputs=2
  Park theta : Subsystem
  Product3 : Product  Multiplication=Matrix(*)  OutDataType=sfix(16)  OutScaling=2^0  RndMeth=Zero
  Selector2 : Selector  InputPortWidth=2  IndexOptions=Index vector (dialog)  Indices=[1]  OutputSizes=1
  Subsystem : Subsystem
  Sum1 : Sum  Inputs=+++|  OutDataType=sfix(16)  OutScaling=2^0
  Sum2 : Sum  Inputs=-+|  OutDataType=sfix(16)  OutScaling=2^0
  To Workspace1 : ToWorkspace  VariableName=Ilqd  SampleTime=-1  SaveFormat=Array
  To Workspace2 : ToWorkspace  VariableName=Vzqd  SampleTime=-1  SaveFormat=Array
  To Workspace3 : ToWorkspace  VariableName=Vlqd3  SampleTime=-1  SaveFormat=Array
  To Workspace4 : ToWorkspace  VariableName=Vlabc3  SampleTime=-1  SaveFormat=Array
  Transformades : Subsystem
  ControlVabc3 : Outport
  P3 : Outport  Port=2
  wires:
  Constant1/1 -> Discrete-Time Integrator/1, Subsystem/1(omega)  "w"
  Discrete-Time Integrator/1 -> Park theta/1(theta)
  Park theta/1(Park) -> Transformades/1(In1)
  Park theta/2(Parkinv) -> Gain1/1
  Sum2/1 -> Controladors PI/1(e)
  Product3/1 -> Memory/1
  Gain1/1 -> Product3/1
  Sum1/1 -> Product3/2, To Workspace3/1  "vlq"
  Memory/1 -> ControlVabc3/1, Gain2/1
  Calcul Potencia/1(P) -> P3/1
  Transformades/2(Iqd) -> Sum2/1, Subsystem/2(ilqd), Calcul Potencia/2(Ilqd), To Workspace1/1
  Mux1/1 -> Sum2/2
  E3/1 -> Càlcul de consignes/2(E3)
  Constant/1 -> Mux1/2
  Càlcul de consignes/1(iqa3) -> Mux1/1
  Selector2/1 -> Càlcul de consignes/1(vzq3)
  Transformades/1(Vzqd) -> Selector2/1, Sum1/1, Calcul Potencia/1(Vzqd), To Workspace2/1
  Controladors PI/1(vlq') -> Sum1/3
  Vzabc/1 -> Transformades/2(Vzabc3)
  Iabc/1 -> Transformades/3(Iabc3)
  Gain2/1 -> To Workspace4/1
  Subsystem/1(desacoblqd1) -> Sum1/2

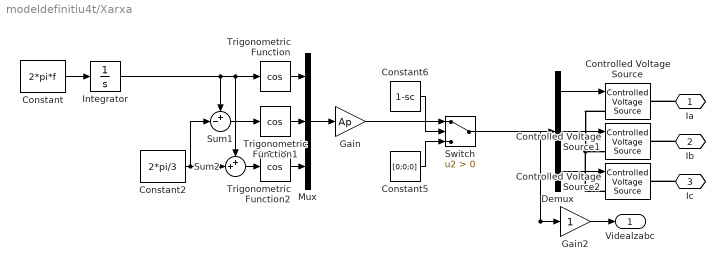
== system modeldefinitiu4t/Xarxa ==
  Constant : Constant  Value=2*pi*f  OutDataType=sfix(16)  OutScaling=2^0
  Constant2 : Constant  Value=2*pi/3  OutDataType=sfix(16)  OutScaling=2^0
  Constant5 : Constant  Value=[0;0;0]  OutDataType=sfix(16)  OutScaling=2^0
  Constant6 : Constant  Value=1-sc  OutDataType=sfix(16)  OutScaling=2^0
  Controlled Voltage Source : powerlib/Electrical Sources/Controlled Voltage Source  DialogController=POWERSYS.PowerSysDialog  SystemSampleTime=-1  Initialize=on  Source_Type=AC  Amplitude=0  Phase=0  Frequency=0  Measurements=None
  Controlled Voltage Source1 : powerlib/Electrical Sources/Controlled Voltage Source  DialogController=POWERSYS.PowerSysDialog  SystemSampleTime=-1  Initialize=on  Source_Type=AC  Amplitude=0  Phase=0  Frequency=0  Measurements=None
  Controlled Voltage Source2 : powerlib/Electrical Sources/Controlled Voltage Source  DialogController=POWERSYS.PowerSysDialog  SystemSampleTime=-1  Initialize=on  Source_Type=AC  Amplitude=0  Phase=0  Frequency=0  Measurements=None
  Demux : Demux  Outputs=3
  Gain : Gain  Gain=Ap  ParameterDataType=sfix(16)  ParameterScaling=2^0  OutDataType=sfix(16)  OutScaling=2^0
  Gain2 : Gain  ParameterDataType=sfix(16)  ParameterScaling=2^0  OutDataType=sfix(16)  OutScaling=2^0  SampleTime=T
  Integrator : Integrator
  Mux : Mux  Inputs=3
  Sum1 : Sum  Inputs=+-|  OutDataType=sfix(16)  OutScaling=2^0
  Sum2 : Sum  Inputs=++|  OutDataType=sfix(16)  OutScaling=2^0
  Switch : Switch  Criteria=u2 > Threshold  OutDataType=sfix(16)  OutScaling=2^0
  Trigonometric Function : Trigonometry  Operator=cos
  Trigonometric Function1 : Trigonometry  Operator=cos
  Trigonometric Function2 : Trigonometry  Operator=cos
  Ia : PMIOPort  Port=1  Side=Left
  Ib : PMIOPort  Port=2  Side=Left
  Ic : PMIOPort  Port=3  Side=Left
  Videalzabc : Outport
  wires:
  Demux/1 -> Controlled Voltage Source/1
  Demux/2 -> Controlled Voltage Source1/1
  Demux/3 -> Controlled Voltage Source2/1
  Constant/1 -> Integrator/1
  Integrator/1 -> Sum1/1, Trigonometric Function/1, Sum2/1
  Sum1/1 -> Trigonometric Function1/1
  Sum2/1 -> Trigonometric Function2/1
  Constant2/1 -> Sum1/2, Sum2/2
  Trigonometric Function/1 -> Mux/1
  Trigonometric Function1/1 -> Mux/2
  Trigonometric Function2/1 -> Mux/3
  Mux/1 -> Gain/1
  Gain/1 -> Switch/1
  Constant5/1 -> Switch/3
  Constant6/1 -> Switch/2
  Gain2/1 -> Videalzabc/1
  Switch/1 -> Gain2/1, Demux/1
  connections:
  Controlled Voltage Source/LConn1 -- Controlled Voltage Source2/LConn1 -- Controlled Voltage Source1/LConn1
  Ia/RConn1 -- Controlled Voltage Source/RConn1
  Ib/RConn1 -- Controlled Voltage Source1/RConn1
  Ic/RConn1 -- Controlled Voltage Source2/RConn1

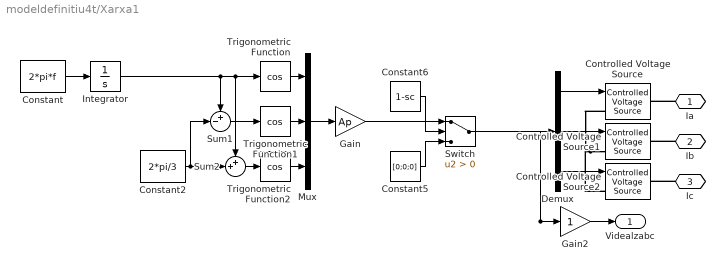
== system modeldefinitiu4t/Xarxa1 ==
  Constant : Constant  Value=2*pi*f  OutDataType=sfix(16)  OutScaling=2^0
  Constant2 : Constant  Value=2*pi/3  OutDataType=sfix(16)  OutScaling=2^0
  Constant5 : Constant  Value=[0;0;0]  OutDataType=sfix(16)  OutScaling=2^0
  Constant6 : Constant  Value=1-sc  OutDataType=sfix(16)  OutScaling=2^0
  Controlled Voltage Source : powerlib/Electrical Sources/Controlled Voltage Source  DialogController=POWERSYS.PowerSysDialog  SystemSampleTime=-1  Initialize=on  Source_Type=AC  Amplitude=0  Phase=0  Frequency=0  Measurements=None
  Controlled Voltage Source1 : powerlib/Electrical Sources/Controlled Voltage Source  DialogController=POWERSYS.PowerSysDialog  SystemSampleTime=-1  Initialize=on  Source_Type=AC  Amplitude=0  Phase=0  Frequency=0  Measurements=None
  Controlled Voltage Source2 : powerlib/Electrical Sources/Controlled Voltage Source  DialogController=POWERSYS.PowerSysDialog  SystemSampleTime=-1  Initialize=on  Source_Type=AC  Amplitude=0  Phase=0  Frequency=0  Measurements=None
  Demux : Demux  Outputs=3
  Gain : Gain  Gain=Ap  ParameterDataType=sfix(16)  ParameterScaling=2^0  OutDataType=sfix(16)  OutScaling=2^0
  Gain2 : Gain  ParameterDataType=sfix(16)  ParameterScaling=2^0  OutDataType=sfix(16)  OutScaling=2^0  SampleTime=T
  Integrator : Integrator
  Mux : Mux  Inputs=3
  Sum1 : Sum  Inputs=+-|  OutDataType=sfix(16)  OutScaling=2^0
  Sum2 : Sum  Inputs=++|  OutDataType=sfix(16)  OutScaling=2^0
  Switch : Switch  Criteria=u2 > Threshold  OutDataType=sfix(16)  OutScaling=2^0
  Trigonometric Function : Trigonometry  Operator=cos
  Trigonometric Function1 : Trigonometry  Operator=cos
  Trigonometric Function2 : Trigonometry  Operator=cos
  Ia : PMIOPort  Port=1  Side=Left
  Ib : PMIOPort  Port=2  Side=Left
  Ic : PMIOPort  Port=3  Side=Left
  Videalzabc : Outport
  wires:
  Gain2/1 -> Videalzabc/1
  Switch/1 -> Demux/1, Gain2/1
  Constant6/1 -> Switch/2
  Constant5/1 -> Switch/3
  Gain/1 -> Switch/1
  Mux/1 -> Gain/1
  Trigonometric Function2/1 -> Mux/3
  Trigonometric Function1/1 -> Mux/2
  Trigonometric Function/1 -> Mux/1
  Constant2/1 -> Sum2/2, Sum1/2
  Sum2/1 -> Trigonometric Function2/1
  Sum1/1 -> Trigonometric Function1/1
  Integrator/1 -> Sum2/1, Trigonometric Function/1, Sum1/1
  Constant/1 -> Integrator/1
  Demux/3 -> Controlled Voltage Source2/1
  Demux/2 -> Controlled Voltage Source1/1
  Demux/1 -> Controlled Voltage Source/1
  connections:
  Ic/RConn1 -- Controlled Voltage Source2/RConn1
  Ib/RConn1 -- Controlled Voltage Source1/RConn1
  Ia/RConn1 -- Controlled Voltage Source/RConn1
  Controlled Voltage Source1/LConn1 -- Controlled Voltage Source2/LConn1 -- Controlled Voltage Source/LConn1

== system modeldefinitiu4t/Subsystem3/Calcul Potencia ==
  Vzqd : Inport
  Ilqd : Inport  Port=2
  Demux2 : Demux  Outputs=2
  Demux3 : Demux  Outputs=2
  Gain9 : Gain  Gain=3/2  ParameterDataType=sfix(16)  ParameterScaling=2^0  OutDataType=sfix(16)  OutScaling=2^0  SampleTime=T
  Product4 : Product  OutDataType=fixdt(1, 16)  OutScaling=2^0  RndMeth=Zero
  Product5 : Product  OutDataType=fixdt(1, 16)  OutScaling=2^0  RndMeth=Zero
  Sum3 : Sum  OutDataType=sfix(16)  OutScaling=2^0
  To Workspace2 : ToWorkspace  VariableName=Pout2  SampleTime=-1  SaveFormat=Array
  P : Outport
  wires:
  Gain9/1 -> To Workspace2/1, P/1
  Ilqd/1 -> Demux3/1
  Vzqd/1 -> Demux2/1
  Demux3/2 -> Product5/2
  Demux3/1 -> Product4/2
  Sum3/1 -> Gain9/1
  Product5/1 -> Sum3/2
  Product4/1 -> Sum3/1
  Demux2/2 -> Product5/1
  Demux2/1 -> Product4/1

== system modeldefinitiu4t/Subsystem3/Controladors PI ==
  e : Inport
  Demux1 : Demux  Outputs=2
  Discrete Zero-Pole : DiscreteZeroPole  Zeros=[-(-Kp+T/2*Ki)/(Kp+T/2*Ki)]  Poles=[1]  Gain=Kp+T/2*Ki  SampleTime=T
  Discrete Zero-Pole1 : DiscreteZeroPole  Zeros=[-(-Kp+T/2*Ki)/(Kp+T/2*Ki)]  Poles=[1]  Gain=Kp+T/2*Ki  SampleTime=T
  Mux2 : Mux  Inputs=2
  vlq' : Outport
  wires:
  Demux1/2 -> Discrete Zero-Pole1/1
  Demux1/1 -> Discrete Zero-Pole/1
  Discrete Zero-Pole/1 -> Mux2/1
  Mux2/1 -> vlq'/1
  e/1 -> Demux1/1
  Discrete Zero-Pole1/1 -> Mux2/2

== system modeldefinitiu4t/Subsystem3/Càlcul de consignes ==
  note: P
  vzq4 : Inport
  E4 : Inport  Port=2
  Constant : Constant  Value=E0  OutDataType=fixdt(1, 16)  OutScaling=2^0
  Divide1 : Product  Inputs=*/  OutDataType=fixdt(1, 16)  OutScaling=2^-10
  Gain : Gain  Gain=K4  ParameterDataType=fixdt(1, 16)  ParameterScaling=2^0  OutDataType=fixdt(1, 16)  OutScaling=2^0
  Gain1 : Gain  Gain=2/3  ParameterDataType=fixdt(1, 16)  ParameterScaling=2^0  OutDataType=fixdt(1, 16)  OutScaling=2^0
  Gain2 : Gain  ParameterDataType=fixdt(1, 16)  ParameterScaling=2^0  OutDataType=fixdt(1, 16)  OutScaling=2^0  SampleTime=T
  Gain6 : Gain  ParameterDataType=fixdt(1, 16)  ParameterScaling=2^0  OutDataType=fixdt(1, 16)  OutScaling=2^0  SampleTime=T
  Gain7 : Gain  ParameterDataType=fixdt(1, 16)  ParameterScaling=2^0  OutDataType=fixdt(1, 16)  OutScaling=2^0  SampleTime=T
  Product : Product  OutDataType=fixdt(1, 16)  OutScaling=2^0  RndMeth=Zero
  Sum : Sum  Inputs=|+-  OutDataType=fixdt(1, 16)  OutScaling=2^0
  iqa4 : Outport
  wires:
  Gain2/1 -> Divide1/2
  E4/1 -> Gain6/1
  Divide1/1 -> iqa4/1  "iq*"
  vzq4/1 -> Gain2/1
  Gain1/1 -> Divide1/1  "P"
  Gain7/1 -> Sum/2
  Gain6/1 -> Product/1, Sum/1
  Gain/1 -> Product/2
  Product/1 -> Gain1/1
  Sum/1 -> Gain/1
  Constant/1 -> Gain7/1

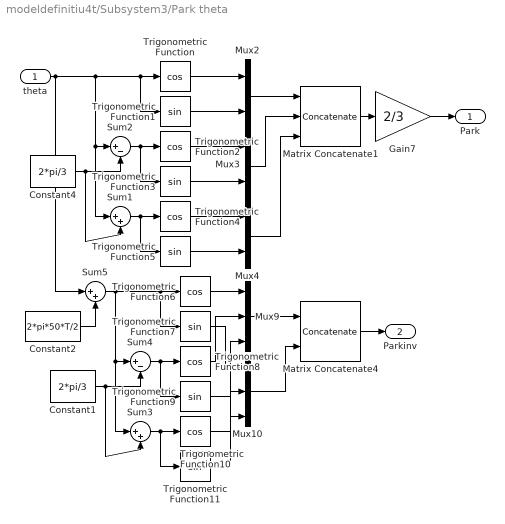
== system modeldefinitiu4t/Subsystem3/Park theta ==
  theta : Inport  PortDimensions=1  OutDataType=sfix(16)  OutScaling=2^0
  Constant1 : Constant  Value=2*pi/3  OutDataType=sfix(16)  OutScaling=2^0  SampleTime=T
  Constant2 : Constant  Value=2*pi*50*T/2  OutDataType=sfix(16)  OutScaling=2^0  SampleTime=T
  Constant4 : Constant  Value=2*pi/3  OutDataType=sfix(16)  OutScaling=2^0  SampleTime=T
  Gain7 : Gain  Gain=2/3  ParameterDataType=sfix(16)  ParameterScaling=2^0  OutDataType=sfix(16)  OutScaling=2^0
  Matrix Concatenate1 : Concatenate  NumInputs=3  Mode=Multidimensional array  ConcatenateDimension=2
  Matrix Concatenate4 : Concatenate  Mode=Multidimensional array  ConcatenateDimension=2
  Mux10 : Mux  Inputs=3
  Mux2 : Mux  Inputs=2
  Mux3 : Mux  Inputs=2
  Mux4 : Mux  Inputs=2
  Mux9 : Mux  Inputs=3
  Sum1 : Sum  Inputs=|++  OutDataType=sfix(16)  OutScaling=2^0
  Sum2 : Sum  Inputs=|+-  OutDataType=sfix(16)  OutScaling=2^0
  Sum3 : Sum  Inputs=|++  OutDataType=sfix(16)  OutScaling=2^0
  Sum4 : Sum  Inputs=|+-  OutDataType=sfix(16)  OutScaling=2^0
  Sum5 : Sum  Inputs=|++  OutDataType=sfix(16)  OutScaling=2^0
  Trigonometric Function{,2,4,6,8,10} (6 alike) : Trigonometry  Operator=cos
  Trigonometric Function{1,3,5,7,9,11} (6 alike) : Trigonometry
  Park : Outport  OutDataType=sfix(16)  OutScaling=2^0
  Parkinv : Outport  Port=2  OutDataType=sfix(16)  OutScaling=2^0
  wires:
  Constant2/1 -> Sum5/2
  Matrix Concatenate4/1 -> Parkinv/1
  Mux10/1 -> Matrix Concatenate4/2
  Mux9/1 -> Matrix Concatenate4/1
  Trigonometric Function11/1 -> Mux10/3
  Trigonometric Function10/1 -> Mux9/3
  Trigonometric Function9/1 -> Mux10/2
  Trigonometric Function8/1 -> Mux9/2
  Trigonometric Function7/1 -> Mux10/1
  Trigonometric Function6/1 -> Mux9/1
  Constant1/1 -> Sum4/2, Sum3/2
  Sum3/1 -> Trigonometric Function10/1, Trigonometric Function11/1
  Sum4/1 -> Trigonometric Function8/1, Trigonometric Function9/1
  Sum5/1 -> Sum3/1, Sum4/1, Trigonometric Function6/1, Trigonometric Function7/1
  Gain7/1 -> Park/1
  Matrix Concatenate1/1 -> Gain7/1
  Mux4/1 -> Matrix Concatenate1/3
  Mux3/1 -> Matrix Concatenate1/2
  Mux2/1 -> Matrix Concatenate1/1
  Trigonometric Function5/1 -> Mux4/2
  Trigonometric Function4/1 -> Mux4/1
  Trigonometric Function3/1 -> Mux3/2
  Trigonometric Function2/1 -> Mux3/1
  Trigonometric Function1/1 -> Mux2/2
  Trigonometric Function/1 -> Mux2/1
  Constant4/1 -> Sum1/2, Sum2/2
  Sum1/1 -> Trigonometric Function5/1, Trigonometric Function4/1
  Sum2/1 -> Trigonometric Function3/1, Trigonometric Function2/1
  theta/1 -> Sum5/1, Trigonometric Function1/1, Trigonometric Function/1, Sum2/1, Sum1/1

== system modeldefinitiu4t/Subsystem3/Subsystem ==
  omega : Inport
  ilqd : Inport  Port=2
  Demux2 : Demux  Outputs=2
  Gain2 : Gain  Gain=Ll  ParameterDataType=sfix(16)  ParameterScaling=2^0  OutDataType=sfix(16)  OutScaling=2^0  SampleTime=T
  Gain3 : Gain  Gain=-Ll  ParameterDataType=sfix(16)  ParameterScaling=2^0  OutDataType=sfix(16)  OutScaling=2^0  SampleTime=T
  Mux1 : Mux  Inputs=2
  Product : Product  OutDataType=fixdt(1, 16)  OutScaling=2^0  RndMeth=Zero
  Product3 : Product  OutDataType=fixdt(1, 16)  OutScaling=2^0  RndMeth=Zero
  desacoblqd1 : Outport
  wires:
  Mux1/1 -> desacoblqd1/1
  Product/1 -> Mux1/2
  Product3/1 -> Mux1/1
  Demux2/1 -> Gain3/1
  Demux2/2 -> Gain2/1
  ilqd/1 -> Demux2/1
  omega/1 -> Product/2, Product3/1
  Gain3/1 -> Product/1
  Gain2/1 -> Product3/2

== system modeldefinitiu4t/Subsystem3/Transformades ==
  In1 : Inport
  Vzabc : Inport  Port=2
  Iabc : Inport  Port=3
  Gain2 : Gain  ParameterDataType=sfix(16)  ParameterScaling=2^0  OutDataType=sfix(16)  OutScaling=2^0  SampleTime=T
  Gain3 : Gain  ParameterDataType=sfix(16)  ParameterScaling=2^0  OutDataType=sfix(16)  OutScaling=2^0  SampleTime=T
  Gain4 : Gain  ParameterDataType=sfix(16)  ParameterScaling=2^0  OutDataType=sfix(16)  OutScaling=2^0  SampleTime=T
  Product1 : Product  Multiplication=Matrix(*)  OutDataType=sfix(16)  OutScaling=2^0  RndMeth=Zero
  Product2 : Product  Multiplication=Matrix(*)  OutDataType=sfix(16)  OutScaling=2^0  RndMeth=Zero
  To Workspace1 : ToWorkspace  VariableName=Ilabc4  SampleTime=-1  SaveFormat=Array
  To Workspace2 : ToWorkspace  VariableName=Vzabc4  SampleTime=-1  SaveFormat=Array
  Vzqd4 : Outport
  Iqd4 : Outport  Port=2
  wires:
  Gain3/1 -> Iqd4/1
  Gain2/1 -> Vzqd4/1
  In1/1 -> Gain4/1
  Product2/1 -> Gain3/1
  Gain4/1 -> Product2/1, Product1/1
  Product1/1 -> Gain2/1
  Iabc/1 -> To Workspace1/1, Product2/2
  Vzabc/1 -> To Workspace2/1, Product1/2

== system modeldefinitiu4t/Subsystem5/Calcul Potencia ==
  Vzqd : Inport
  Ilqd : Inport  Port=2
  Demux2 : Demux  Outputs=2
  Demux3 : Demux  Outputs=2
  Gain9 : Gain  Gain=3/2  ParameterDataType=sfix(16)  ParameterScaling=2^0  OutDataType=sfix(16)  OutScaling=2^0  SampleTime=T
  Product4 : Product  OutDataType=fixdt(1, 16)  OutScaling=2^0  RndMeth=Zero
  Product5 : Product  OutDataType=fixdt(1, 16)  OutScaling=2^0  RndMeth=Zero
  Sum3 : Sum  OutDataType=sfix(16)  OutScaling=2^0
  To Workspace2 : ToWorkspace  VariableName=Pout1  SampleTime=-1  SaveFormat=Array
  P : Outport
  wires:
  Demux2/1 -> Product4/1
  Demux2/2 -> Product5/1
  Product4/1 -> Sum3/1
  Product5/1 -> Sum3/2
  Sum3/1 -> Gain9/1
  Demux3/1 -> Product4/2
  Demux3/2 -> Product5/2
  Vzqd/1 -> Demux2/1
  Ilqd/1 -> Demux3/1
  Gain9/1 -> P/1, To Workspace2/1

== system modeldefinitiu4t/Subsystem5/Controladors PI ==
  e : Inport
  Demux1 : Demux  Outputs=2
  Discrete Zero-Pole : DiscreteZeroPole  Zeros=[-(-Kp+T/2*Ki)/(Kp+T/2*Ki)]  Poles=[1]  Gain=Kp+T/2*Ki  SampleTime=T
  Discrete Zero-Pole1 : DiscreteZeroPole  Zeros=[-(-Kp+T/2*Ki)/(Kp+T/2*Ki)]  Poles=[1]  Gain=Kp+T/2*Ki  SampleTime=T
  Mux2 : Mux  Inputs=2
  vlq' : Outport
  wires:
  Discrete Zero-Pole1/1 -> Mux2/2
  e/1 -> Demux1/1
  Mux2/1 -> vlq'/1
  Discrete Zero-Pole/1 -> Mux2/1
  Demux1/1 -> Discrete Zero-Pole/1
  Demux1/2 -> Discrete Zero-Pole1/1
